simulink model "Infrastructure_Server"  (R2023b)
settings: Solver=FixedStepDiscrete  StartTime=0.0  StopTime=inf  FixedStep=0.002  RelTol=1e-3  EnableMultiTasking=on
undefined symbols (not defined in the file or in its folder): DiscIntNeverNeededParam, qc_get_step_size
libraries: quarc_library x11
settings Model: ExtModeTrigDuration=10000  Creator=PK  LastModifiedBy=PK
settings SolverCC: AlgebraicLoopSolver=TrustRegion  PositivePriorityOrder=on
settings DataIOCC: ReturnWorkspaceOutputs=off
settings DebuggingCC: UnconnectedInputMsg=warning  UnconnectedOutputMsg=warning  UnconnectedLineMsg=warning  ArithmeticOperatorsInVariantConditions=warning
settings ModelReferenceCC: EnableRefExpFcnMdlSchedulingChecks=on
settings SFSimCC: SimUseLocalCustomCode=off  CustomCodeUndefinedFunction=UseInterfaceOnly
settings RTWCC: Description=QUARC Win64 Target Using Toolchain  SystemTargetFile=quarc_win64.tlc  TemplateMakefile=quarc_default_tmf  RTWUseLocalCustomCode=off  Toolchain=QUARC win64 | nmake (64-bit Windows)  BuildConfiguration=Faster Runs
settings CodeAppCC: StateflowObjectComments=on
settings STFCustomTargetCC: ConcurrentExecutionCompliant=on  GRTInterface=on  UseToolchainInfoCompliant=on  SystemTargetFile=quarc_win64.tlc
settings GRTTargetCC: ParMdlRefBuildCompliant=off  CompOptLevelCompliant=off  CombineOutputUpdateFcns=off  MatFileLogging=off  CPPClassGenCompliant=off  GRTInterface=on  ExtMode=on  ExtModeMexFile=quarc_comm
settings ConfigComp: CovMetricSettings=dswe

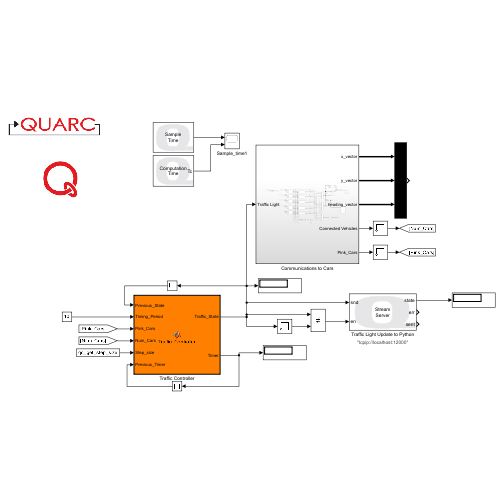
[thumbnail: Simulink's stored preview of the top-level diagram]
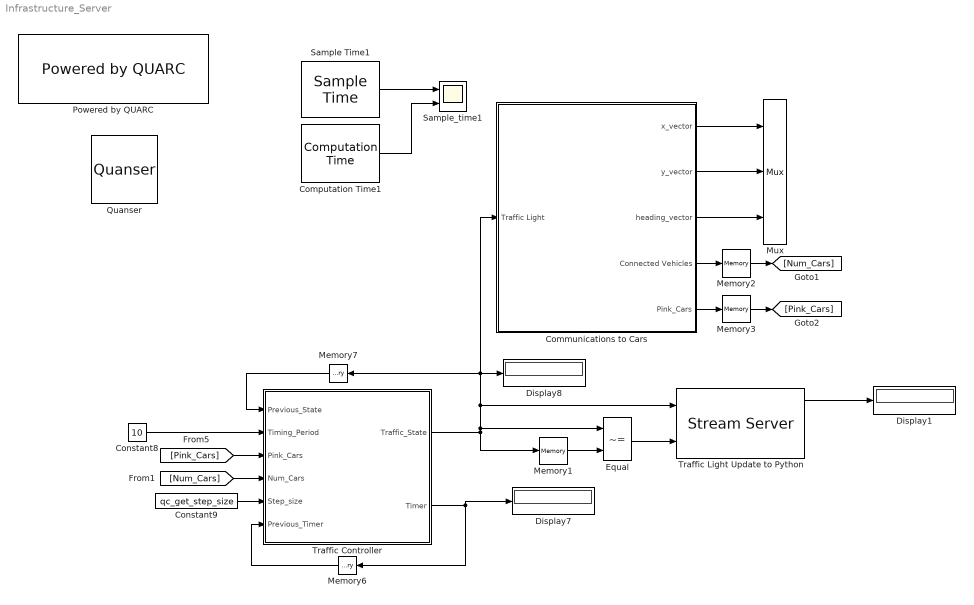
== system Infrastructure_Server ==
  Communications to Cars : Subsystem
  Computation Time1 : quarc_library/Sources/Time/Computation Time  sample_time=qc_get_step_size  use_model=on  use_cpu_time=off
  Constant8 : Constant  Value=10
  Constant9 : Constant  Value=qc_get_step_size
  Display1 : Display
  Display7 : Display
  Display8 : Display
  Equal : RelationalOperator  Operator=~=  OutDataTypeStr=boolean  RndMeth=Simplest  InputSameDT=off
  Memory1 : Memory
  Memory2 : Memory  InheritSampleTime=on  LinearizeMemory=on  LinearizeAsDelay=on
  Memory3 : Memory  InheritSampleTime=on  LinearizeMemory=on  LinearizeAsDelay=on
  Memory6 : Memory  InheritSampleTime=on  LinearizeMemory=on  LinearizeAsDelay=on
  Memory7 : Memory  InitialCondition=1  InheritSampleTime=on  LinearizeMemory=on  LinearizeAsDelay=on
  Mux : Mux  Inputs=3
  Powered by QUARC : quarc_library/Logos/Powered by QUARC
  Quanser : quarc_library/Logos/Quanser
  Sample Time1 : quarc_library/Sources/Time/Sample Time  Priority=-99  sample_time=qc_get_step_size
  Sample_time1 : Scope  NumInputPorts=2
  Traffic Controller : MATLAB Function  TreatAsAtomicUnit=on
  Traffic Light Update to Python : quarc_library/Communications/Basic/Stream Server  uri_source=Specify via dialog (do not evaluate)  uri=tcpip://localhost:12000  send_buffer_size=1460  receive_buffer_size=1460  byte_order=little endian (Intel - LSB first)  optimization=Minimum latency  send_options=Send most recent data  receive_options=Do not receive data  default_value=[5 5]  sample_time=-1  active=off  implementation=Use blocking I/O in a separate thread  send_fifo_size=1000  receive_fifo_size=1000  send_priority=0  receive_priority=0  send_dimensions=off  receive_dimensions=off  max_dimensions=-1  data_type=Inherited via back propagation  type_expr=BusObject
      settings: AttributesFormatString="\"tcpip://localhost:12000\""
  wires:
  Equal/1 -> Traffic Light Update to Python/2
  Constant9/1 -> Traffic Controller/5(Step_size)
  Memory3/1 -> [Pink_Cars]
  Memory1/1 -> Equal/2
  Memory2/1 -> [Num_Cars]
  Communications to Cars/2(y_vector) -> Mux/2
  [Num_Cars] -> Traffic Controller/4(Num_Cars)
  Communications to Cars/4(Connected Vehicles) -> Memory2/1
  Traffic Controller/1(Traffic_State) -> Display8/1, Communications to Cars/1(Traffic Light), Memory7/1, Traffic Light Update to Python/1, Equal/1, Memory1/1
  Communications to Cars/5(Pink_Cars) -> Memory3/1
  Sample Time1/1 -> Sample_time1/1
  [Pink_Cars] -> Traffic Controller/3(Pink_Cars)
  Communications to Cars/3(heading_vector) -> Mux/3
  Constant8/1 -> Traffic Controller/2(Timing_Period)
  Computation Time1/1 -> Sample_time1/2
  Memory6/1 -> Traffic Controller/6(Previous_Timer)
  Memory7/1 -> Traffic Controller/1(Previous_State)
  Traffic Light Update to Python/1 -> Display1/1
  Communications to Cars/1(x_vector) -> Mux/1
  Traffic Controller/2(Timer) -> Display7/1, Memory6/1

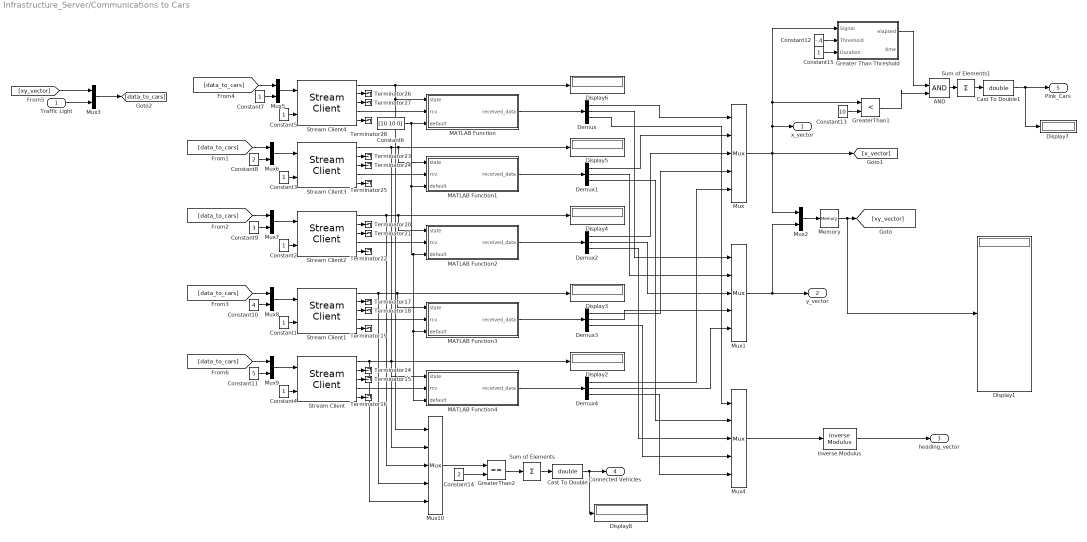
== system Infrastructure_Server/Communications to Cars ==
  Traffic Light : Inport
  AND : Logic  IconShape=distinctive  AllPortsSameDT=off  OutDataTypeStr=boolean
  Cast To Double : DataTypeConversion  OutDataTypeStr=double  SaturateOnIntegerOverflow=off  RndMeth=Floor
  Cast To Double1 : DataTypeConversion  OutDataTypeStr=double  SaturateOnIntegerOverflow=off  RndMeth=Floor
  Constant{1..5,7,15} (7 alike) : Constant
  Constant10 : Constant  Value=4
  Constant11 : Constant  Value=5
  Constant12 : Constant  Value=-.4
  Constant13 : Constant  Value=10
  Constant14 : Constant  Value=2
  Constant6 : Constant  Value=[10 10 0]
  Constant8 : Constant  Value=2
  Constant9 : Constant  Value=3
  Demux{,1..4} (5 alike) : Demux  Outputs=3
  Display{1..8} (8 alike) : Display
      settings: Decimation=100
  Greater Than Threshold : Subsystem
  GreaterThan1 : RelationalOperator  Operator=<  OutDataTypeStr=boolean  RndMeth=Simplest  InputSameDT=off
  GreaterThan2 : RelationalOperator  Operator===  OutDataTypeStr=boolean  RndMeth=Simplest  InputSameDT=off
  Inverse Modulus : quarc_library/Discontinuities/Inverse Modulus  modulus=2*pi  output_derivative=off  output_revolutions=off  max_x=Inf  min_x=-Inf
  MATLAB Function : MATLAB Function  TreatAsAtomicUnit=on
  MATLAB Function1 : MATLAB Function  TreatAsAtomicUnit=on
  MATLAB Function2 : MATLAB Function  TreatAsAtomicUnit=on
  MATLAB Function3 : MATLAB Function  TreatAsAtomicUnit=on
  MATLAB Function4 : MATLAB Function  TreatAsAtomicUnit=on
  Memory : Memory  InitialCondition=10*ones(1,10)  InheritSampleTime=on  LinearizeMemory=on  LinearizeAsDelay=on
  Mux{,1,4,10} (4 alike) : Mux  Inputs=5
  Mux{2..3,5..9} (7 alike) : Mux  Inputs=2
  Stream Client : quarc_library/Communications/Basic/Stream Client  uri_source=Specify via dialog (do not evaluate)  uri=tcpip://localhost:5555?nagle='off'  send_buffer_size=1460  receive_buffer_size=1460  byte_order=little endian (Intel - LSB first)  optimization=Minimum latency  send_options=Send most recent data  receive_options=Receive most recent data  default_value=[10 10 0]  sample_time=qc_get_step_size  active=off  implementation=Use blocking I/O in a separate thread  send_fifo_size=1  receive_fifo_size=1  send_priority=0  receive_priority=0  send_dimensions=off  receive_dimensions=off  max_dimensions=-1  data_type=Inherited via back propagation  type_expr=BusObject
      settings: AttributesFormatString="\"tcpip://localhost:5555?nagle='off'\""
  Stream Client1 : quarc_library/Communications/Basic/Stream Client  uri_source=Specify via dialog (do not evaluate)  uri=tcpip://localhost:4444?nagle='off'  send_buffer_size=1460  receive_buffer_size=1460  byte_order=little endian (Intel - LSB first)  optimization=Minimum latency  send_options=Send most recent data  receive_options=Receive most recent data  default_value=[10 10 0]  sample_time=qc_get_step_size  active=off  implementation=Use blocking I/O in a separate thread  send_fifo_size=1  receive_fifo_size=1  send_priority=0  receive_priority=0  send_dimensions=off  receive_dimensions=off  max_dimensions=-1  data_type=Inherited via back propagation  type_expr=BusObject
      settings: AttributesFormatString="\"tcpip://localhost:4444?nagle='off'\""
  Stream Client2 : quarc_library/Communications/Basic/Stream Client  uri_source=Specify via dialog (do not evaluate)  uri=tcpip://localhost:3333?nagle='off'  send_buffer_size=1460  receive_buffer_size=1460  byte_order=little endian (Intel - LSB first)  optimization=Minimum latency  send_options=Send most recent data  receive_options=Receive most recent data  default_value=[10 10 0]  sample_time=qc_get_step_size  active=off  implementation=Use blocking I/O in a separate thread  send_fifo_size=1  receive_fifo_size=1  send_priority=0  receive_priority=0  send_dimensions=off  receive_dimensions=off  max_dimensions=-1  data_type=Inherited via back propagation  type_expr=BusObject
      settings: AttributesFormatString="\"tcpip://localhost:3333?nagle='off'\""
  Stream Client3 : quarc_library/Communications/Basic/Stream Client  uri_source=Specify via dialog (do not evaluate)  uri=tcpip://localhost:2222?nagle='off'  send_buffer_size=1460  receive_buffer_size=1460  byte_order=little endian (Intel - LSB first)  optimization=Minimum latency  send_options=Send most recent data  receive_options=Receive most recent data  default_value=[10 10 0]  sample_time=qc_get_step_size  active=off  implementation=Use blocking I/O in a separate thread  send_fifo_size=1  receive_fifo_size=1  send_priority=0  receive_priority=0  send_dimensions=off  receive_dimensions=off  max_dimensions=-1  data_type=Inherited via back propagation  type_expr=BusObject
      settings: AttributesFormatString="\"tcpip://localhost:2222?nagle='off'\""
  Stream Client4 : quarc_library/Communications/Basic/Stream Client  uri_source=Specify via dialog (do not evaluate)  uri=tcpip://localhost:1111?nagle='off'  send_buffer_size=1460  receive_buffer_size=1460  byte_order=little endian (Intel - LSB first)  optimization=Minimum latency  send_options=Send most recent data  receive_options=Receive most recent data  default_value=[10 10 0]  sample_time=qc_get_step_size  active=off  implementation=Use blocking I/O in a separate thread  send_fifo_size=1  receive_fifo_size=1  send_priority=0  receive_priority=0  send_dimensions=off  receive_dimensions=off  max_dimensions=-1  data_type=Inherited via back propagation  type_expr=BusObject
      settings: AttributesFormatString="\"tcpip://localhost:1111?nagle='off'\""
  Sum of Elements : Sum  Inputs=+
  Sum of Elements1 : Sum  Inputs=+
  Terminator{14..28} (15 alike) : Terminator
  x_vector : Outport
  y_vector : Outport  Port=2
  heading_vector : Outport  Port=3
  Connected Vehicles : Outport  Port=4
  Pink_Cars : Outport  Port=5
  wires:
  Demux4/1 -> Mux/5
  Demux1/1 -> Mux/2
  Demux/1 -> Mux/1
  Stream Client1/5 -> Terminator19/1
  Stream Client4/1 -> MATLAB Function/1(state), Mux10/1, Display6/1
  Stream Client2/3 -> Terminator21/1
  Stream Client2/2 -> Terminator20/1
  Stream Client1/3 -> Terminator18/1
  MATLAB Function4/1(received_data) -> Demux4/1
  Stream Client3/3 -> Terminator24/1
  Demux2/1 -> Mux/3
  Stream Client1/2 -> Terminator17/1
  Memory/1 -> Display1/1, [xy_vector]
  Constant4/1 -> Stream Client/2
  Stream Client4/5 -> Terminator28/1
  Stream Client/1 -> MATLAB Function4/1(state), Display2/1, Mux10/5
  Stream Client3/1 -> Mux10/2, MATLAB Function1/1(state), Display5/1
  Constant3/1 -> Stream Client3/2
  Stream Client1/1 -> Mux10/4, MATLAB Function3/1(state), Display3/1
  Constant5/1 -> Stream Client4/2
  MATLAB Function/1(received_data) -> Demux/1
  Mux/1 -> Greater Than Threshold/1(Signal), GreaterThan1/1, x_vector/1, Mux2/1, [x_vector]
  Stream Client4/2 -> Terminator26/1
  Mux1/1 -> y_vector/1, Mux2/2
  Mux2/1 -> Memory/1
  Constant6/1 -> MATLAB Function4/3(default), MATLAB Function3/3(default), MATLAB Function2/3(default), MATLAB Function1/3(default), MATLAB Function/3(default)
  Stream Client2/1 -> Mux10/3, MATLAB Function2/1(state), Display4/1
  MATLAB Function3/1(received_data) -> Demux3/1
  Stream Client/4 -> MATLAB Function4/2(rcv)
  MATLAB Function1/1(received_data) -> Demux1/1
  Demux/2 -> Mux1/1
  Constant2/1 -> Stream Client2/2
  Stream Client2/5 -> Terminator22/1
  MATLAB Function2/1(received_data) -> Demux2/1
  Demux1/2 -> Mux1/2
  Demux3/1 -> Mux/4
  Stream Client3/2 -> Terminator23/1
  Demux2/2 -> Mux1/3
  Stream Client3/4 -> MATLAB Function1/2(rcv)
  Constant1/1 -> Stream Client1/2
  Stream Client2/4 -> MATLAB Function2/2(rcv)
  Stream Client/5 -> Terminator16/1
  Stream Client1/4 -> MATLAB Function3/2(rcv)
  Stream Client4/4 -> MATLAB Function/2(rcv)
  Demux3/2 -> Mux1/4
  Stream Client/2 -> Terminator14/1
  Stream Client/3 -> Terminator15/1
  Stream Client4/3 -> Terminator27/1
  Stream Client3/5 -> Terminator25/1
  [xy_vector] -> Mux3/1
  Mux3/1 -> [data_to_cars]
  Traffic Light/1 -> Mux3/2
  Demux4/2 -> Mux1/5
  Demux4/3 -> Mux4/5
  Demux3/3 -> Mux4/4
  Demux2/3 -> Mux4/3
  Demux1/3 -> Mux4/2
  Demux/3 -> Mux4/1
  Mux4/1 -> Inverse Modulus/1
  Inverse Modulus/1 -> heading_vector/1
  Mux5/1 -> Stream Client4/1
  [data_to_cars] -> Mux5/1
  Constant7/1 -> Mux5/2
  Constant8/1 -> Mux6/2
  [data_to_cars] -> Mux6/1
  [data_to_cars] -> Mux7/1
  Constant9/1 -> Mux7/2
  Constant10/1 -> Mux8/2
  [data_to_cars] -> Mux8/1
  [data_to_cars] -> Mux9/1
  Constant11/1 -> Mux9/2
  Mux6/1 -> Stream Client3/1
  Mux7/1 -> Stream Client2/1
  Mux8/1 -> Stream Client1/1
  Mux9/1 -> Stream Client/1
  AND/1 -> Sum of Elements1/1
  Constant13/1 -> GreaterThan1/2
  GreaterThan1/1 -> AND/2
  Sum of Elements1/1 -> Cast To Double1/1
  Mux10/1 -> GreaterThan2/1
  GreaterThan2/1 -> Sum of Elements/1
  Sum of Elements/1 -> Cast To Double/1
  Constant14/1 -> GreaterThan2/2
  Cast To Double/1 -> Display8/1, Connected Vehicles/1
  Cast To Double1/1 -> Display7/1, Pink_Cars/1
  Greater Than Threshold/1(elapsed) -> AND/1
  Constant12/1 -> Greater Than Threshold/2(Threshold)
  Constant15/1 -> Greater Than Threshold/3(Duration)

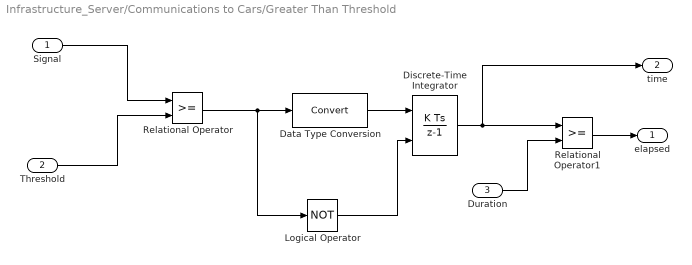
== system Infrastructure_Server/Communications to Cars/Greater Than Threshold ==
  Signal : Inport
  Threshold : Inport  Port=2
  Duration : Inport  Port=3
  Data Type Conversion : DataTypeConversion  SaturateOnIntegerOverflow=off  RndMeth=Floor
  Discrete-Time Integrator : DiscreteIntegrator  Priority=1  ExternalReset=level  SampleTime=qc_get_step_size  ICPrevOutput=DiscIntNeverNeededParam  ICPrevScaledInput=DiscIntNeverNeededParam
  Logical Operator : Logic  Operator=NOT  AllPortsSameDT=off  OutDataTypeStr=boolean
  Relational Operator : RelationalOperator  InputSameDT=off
  Relational Operator1 : RelationalOperator  InputSameDT=off
  elapsed : Outport  VectorParamsAs1DForOutWhenUnconnected=off
  time : Outport  Port=2  VectorParamsAs1DForOutWhenUnconnected=off
  wires:
  Data Type Conversion/1 -> Discrete-Time Integrator/1
  Signal/1 -> Relational Operator/1
  Threshold/1 -> Relational Operator/2
  Relational Operator/1 -> Data Type Conversion/1, Logical Operator/1
  Logical Operator/1 -> Discrete-Time Integrator/2
  Discrete-Time Integrator/1 -> Relational Operator1/1, time/1
  Duration/1 -> Relational Operator1/2
  Relational Operator1/1 -> elapsed/1

== matlab function Infrastructure_Server/Communications to Cars/MATLAB Function1 ==
  data: state input; received_data output; rcv input; default input
function received_data = state_checker (state, rcv, default)
received_data = rcv;
if state == 0
    received_data = default;
end
end

== matlab function Infrastructure_Server/Communications to Cars/MATLAB Function ==
  data: state input; received_data output; rcv input; default input
function received_data = state_checker (state, rcv, default)
received_data = rcv;
if state == 0
    received_data = default;
end
end

== matlab function Infrastructure_Server/Communications to Cars/MATLAB Function2 ==
  data: state input; received_data output; rcv input; default input
function received_data = state_checker (state, rcv, default)
received_data = rcv;
if state == 0
    received_data = default;
end
end

== matlab function Infrastructure_Server/Communications to Cars/MATLAB Function3 ==
  data: state input; received_data output; rcv input; default input
function received_data = state_checker (state, rcv, default)
received_data = rcv;
if state == 0
    received_data = default;
end
end

== matlab function Infrastructure_Server/Communications to Cars/MATLAB Function4 ==
  data: state input; received_data output; rcv input; default input
function received_data = state_checker (state, rcv, default)
received_data = rcv;
if state == 0
    received_data = default;
end
end

== matlab function Infrastructure_Server/Traffic Controller ==
  data: Previous_State input; Timing_Period input; Pink_Cars input; Num_Cars input; Traffic_State output; Step_size input; Previous_Timer input; Timer output
function [Traffic_State, Timer]  = Traffic_Controller (Previous_State, Timing_Period, Pink_Cars, Num_Cars, Step_size, Previous_Timer)
%#codegen
Traffic_State = Previous_State;
Timer = Previous_Timer + Step_size;

if Num_Cars == 0
    Pink_Timing = Timing_Period;
    Blue_Timing = Timing_Period;
    Blue_Cars = -1;
    Pink_Cars = -1;
else
    Blue_Cars = Num_Cars - Pink_Cars;
    Pink_Timing = Pink_Cars/Num_Cars*Timing_Period;
    Blue_Timing =Blue_Cars/Num_Cars*Timing_Period;
end

switch Traffic_State
    % Case 0 - Red Light, Case 1 - Green Light
    
    case 0
        if ((Timer > Blue_Timing) && (Blue_Cars < Num_Cars))
            Traffic_State = 1;
            Timer = 0;
        end
        
    case 1
        if ((Timer > Pink_Timing) && (Pink_Cars < Num_Cars))
            Traffic_State = 0;
            Timer = 0;
        end
        
end
end
